simulink model "SPMe_ESC_validation_simulink"  (R2024a)
settings: Solver=FixedStepAuto  StartTime=0.0  StopTime=t_end  FixedStep=param.dt  MaxStep=1  RelTol=1e-6
values from neighbouring files (symbols this model uses):
  R_esc = R_escs(param.soc_name)    [SPMe_EqCM_ESC_validation.m]    (also in run_SPMe_ESC_validation.m = 0.0067; run_parallel_SPMe_ESC.m = 0.0134)
  R_tab = R_tabs(param.soc_name)    [SPMe_EqCM_ESC_validation.m]    (also in run_SPMe_ESC_validation.m = 0.0086; run_parallel_SPMe_ESC.m = 0.0172)
  V_min = 0    [SPMe_EqCM_ESC_validation.m]    (also in run_SPMe_ESC_validation.m; run_parallel_SPMe_ESC.m)
libraries: eeGeneralControl x1, simulink x1
settings Model: Creator=tom  LastModifiedBy=Vivian
settings SolverCC: AlgebraicLoopSolver=TrustRegion
settings DebuggingCC: UnconnectedInputMsg=warning  UnconnectedOutputMsg=warning  UnconnectedLineMsg=warning
settings ModelReferenceCC: EnableRefExpFcnMdlSchedulingChecks=on
settings RTWCC: GPUComputeCapability=3.5  DLArmComputeVersion=19.05

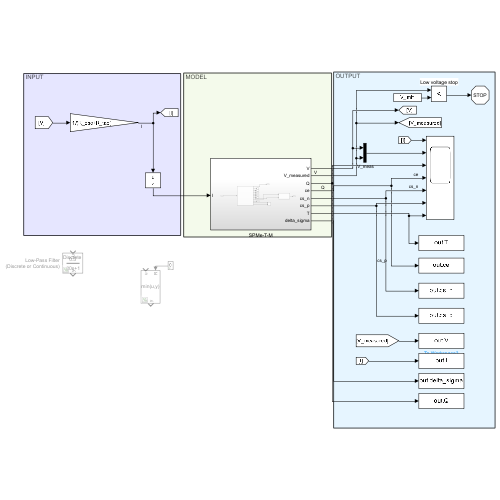
[thumbnail: Simulink's stored preview of the top-level diagram]
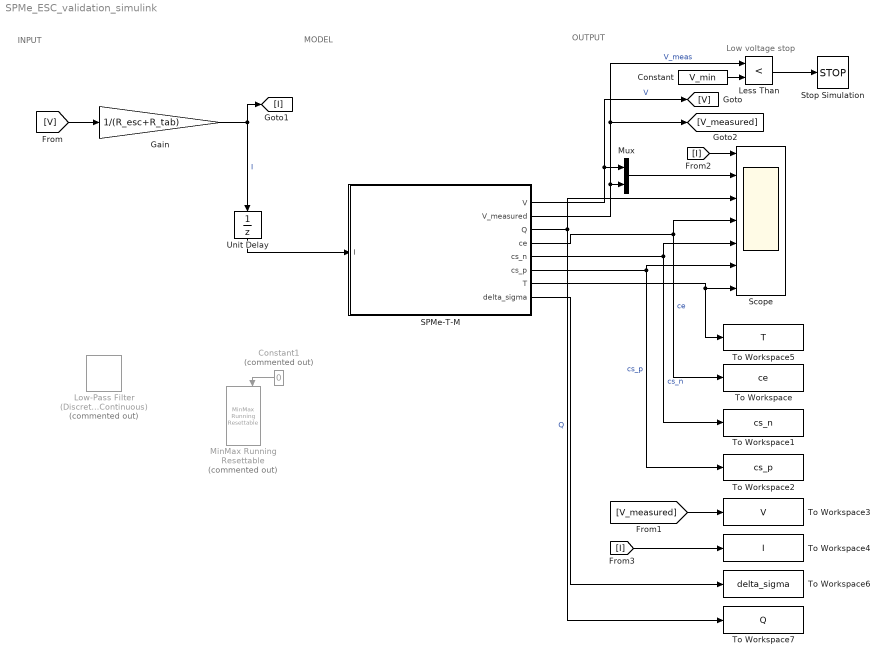
== system SPMe_ESC_validation_simulink ==
  note: OUTPUT
  note: MODEL
  note: INPUT
  note: Low voltage stop
  Constant : Constant  Value=V_min
  Constant1 : Constant  Commented=on  Value=0
  Gain : Gain  Gain=1/(R_esc+R_tab)
  Less Than : RelationalOperator  Operator=<  OutDataTypeStr=boolean  RndMeth=Simplest  InputSameDT=off
  Low-Pass Filter (Discrete or Continuous) : eeGeneralControl/Low-Pass Filter (Discrete or Continuous)  Commented=on  K=0.5  T=20  B=inf  A=-inf  init_option=Inherited from block input  x0=0  Ts=-1
  MinMax Running Resettable : simulink/Math Operations/MinMax Running Resettable  Commented=on  Function=min  vinit=1000
  Mux : Mux  Inputs=2
  SPMe-T-M : Subsystem
  Scope : Scope  NumInputPorts=7
  Stop Simulation : Stop
  To Workspace : ToWorkspace  VariableName=ce  SaveFormat=Timeseries  SampleTime=-1
  To Workspace1 : ToWorkspace  VariableName=cs_n  SaveFormat=Timeseries  SampleTime=-1
  To Workspace2 : ToWorkspace  VariableName=cs_p  SaveFormat=Timeseries  SampleTime=-1
  To Workspace3 : ToWorkspace  VariableName=V  SaveFormat=Timeseries  SampleTime=-1
  To Workspace4 : ToWorkspace  VariableName=I  SaveFormat=Timeseries  SampleTime=-1
  To Workspace5 : ToWorkspace  VariableName=T  SaveFormat=Timeseries  SampleTime=-1
  To Workspace6 : ToWorkspace  VariableName=delta_sigma  SaveFormat=Timeseries  SampleTime=-1
  To Workspace7 : ToWorkspace  VariableName=Q  SaveFormat=Timeseries  SampleTime=-1
  Unit Delay : UnitDelay  SampleTime=-1  HasFrameUpgradeWarning=on
  wires:
  SPMe-T-M/3(Q) -> To Workspace7/1, Scope/3  "Q"
  SPMe-T-M/5(cs_n) -> Scope/5, To Workspace1/1  "cs_n"
  SPMe-T-M/6(cs_p) -> Scope/6, To Workspace2/1  "cs_p"
  Less Than/1 -> Stop Simulation/1
  Constant/1 -> Less Than/2
  SPMe-T-M/4(ce) -> To Workspace/1, Scope/4  "ce"
  SPMe-T-M/1(V) -> [V], Mux/1  "V"
  SPMe-T-M/2(V_measured) -> Less Than/1, [V_measured], Mux/2  "V_meas"
  Gain/1 -> Unit Delay/1, [I]  "I"
  Mux/1 -> Scope/2
  [V_measured] -> To Workspace3/1
  [I] -> Scope/1
  [I] -> To Workspace4/1
  SPMe-T-M/7(T) -> To Workspace5/1, Scope/7
  [V] -> Gain/1
  SPMe-T-M/8(delta_sigma) -> To Workspace6/1
  Unit Delay/1 -> SPMe-T-M/1(I)
  Constant1/1 -> MinMax Running Resettable/2

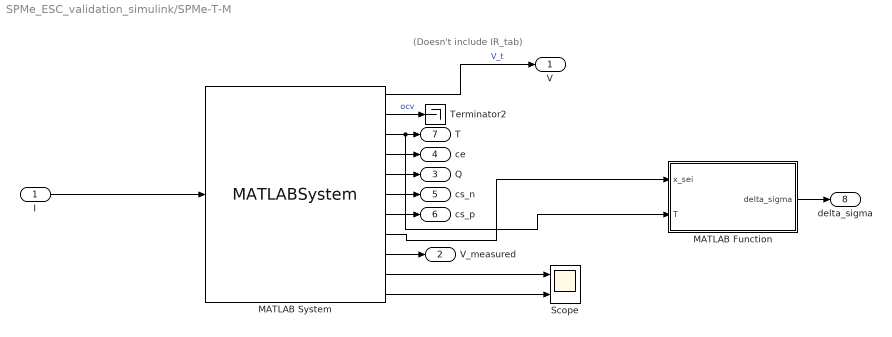
== system SPMe_ESC_validation_simulink/SPMe-T-M ==
  note: (Doesn't include IR_tab)
  I : Inport
  MATLAB Function : MATLAB Function  TreatAsAtomicUnit=on
  MATLAB System : MATLABSystem  System=pybamm_bat  SimulateUsing=Interpreted execution
      mask Type: pybamm_bat
      mask Display:
      | disp('pybamm_bat');
      | port_label('input',1,'current');
      | port_label('output',1,'V_t');
      | port_label('output',2,'ocv');
      | port_label('output',3,'T');
      | port_label('output',4,'ce');
      | port_label('output',5,'heating');
      | port_label('output',6,'neg_conc');
      | port_label('output',7,'pos_conc');
      | port_label('output',8,'x_sei');
      | port_label('output',9,'V_meas');
      | port_label('output',10,'ocp_n');
      | port_label('output',11,'ocp_p');
  Scope : Scope  NumInputPorts=2
  Terminator2 : Terminator
  V : Outport
  V_measured : Outport  Port=2
  Q : Outport  Port=3  VectorParamsAs1DForOutWhenUnconnected=off
  ce : Outport  Port=4
  cs_n : Outport  Port=5  VectorParamsAs1DForOutWhenUnconnected=off
  cs_p : Outport  Port=6  VectorParamsAs1DForOutWhenUnconnected=off
  T : Outport  Port=7
  delta_sigma : Outport  Port=8
  wires:
  MATLAB System/4 -> ce/1
  MATLAB System/5 -> Q/1
  MATLAB System/6 -> cs_n/1
  MATLAB System/7 -> cs_p/1
  MATLAB System/1 -> V/1  "V_t"
  MATLAB System/8 -> MATLAB Function/1(x_sei)
  MATLAB System/9 -> V_measured/1
  MATLAB System/3 -> MATLAB Function/2(T), T/1
  MATLAB System/2 -> Terminator2/1  "ocv"
  MATLAB Function/1(delta_sigma) -> delta_sigma/1
  I/1 -> MATLAB System/1
  MATLAB System/10 -> Scope/1
  MATLAB System/11 -> Scope/2

== matlab function SPMe_ESC_validation_simulink/SPMe-T-M/MATLAB Function ==
  data: x_sei input; delta_sigma output; T input
function delta_sigma  = expansion(x_sei, T)
%XSEI2PTOTAL 
% Mechanical params
M_C6 = 72/1000; %kg/mol
% V_head_0 = 6.65e-6; %m3 (0.121*0.074*0.0055)*0.135
% L = 2.4/1000; %m
% E = 0.19e6; %Pa
% alpha_cell = 1.1e-6; %m/K
% P_atm = 101; %kPa
% P_crit = 158.7731; %kPa
R = 8.3145; %J.mol-1.K-1
A = 0.009; %m2 (0.121*0.074)
DMC = [6.4338; 1413; -44.25]; %Antoine coeffs [A B C] 
EC = [6.4897; 1836.57; -102.23];
y_dmc = 0.7;
y_ec = 1-y_dmc;         
m_an = 0.0191; 
x_sei_0 = 0.15;
% T_amb = 273.15+25; % K
% sigma_0 = 1.5120e+04;

% Internal cell pressure
V_head_0 = 6.65e-06; %m-3
L_p0 = 2.4e-3; %m for 2 poron
E_p = 0.19e6; %Pa Young's modulus for poron
% E_c = 1e12; %assume large by default
alpha = 1.1e-6; %m/K
P_atm = 101e3; %Pa
% P_crit = 158e3; %Pa
% P0 = 14e3; %Pa
R = 8.3145; %J.mol-1.K-1
% k_b = 1.380649e-23; %m2.kg.s-2.K-1;
T_amb = 273.15+25; % K
sigma_0 = 1.5120e+04;
% L_cs0 = 5.5e-3; %m initial cell solid thickness
% V_cell = 0.130*0.089*0.055; % [130mm×89mm×5.5mm] active material

% P_elyte
Psat_EC = 10.^(EC(1)-EC(2)./(EC(3)+T));
Psat_DMC = 10.^(DMC(1)-DMC(2)./(DMC(3)+T)); 
P_elyte = (y_dmc*Psat_DMC + y_ec*Psat_EC)*1e3; 

% P_CO2
n_CO2 = 0.5*m_an/M_C6*(x_sei_0-x_sei);

% Solve for gas volume and pressure
delta_sigma_calc = P_elyte - sigma_0 - P_atm;
a = 1;
b = -(V_head_0 + A.*(L_p0/E_p*(delta_sigma_calc) - alpha.*(T-T_amb)));
c = -A*L_p0/E_p.*n_CO2.*R.*(T);
V_g0 = (-b+sqrt(max(b.^2-4.*a.*c,0)))/(2*a);
V_g = max(V_g0, V_head_0); % min V_g = V_head_0

P_CO2 = n_CO2.*R.*T./V_g;
P_gas = P_elyte + P_CO2;

delta_sigma = max(P_gas-P_atm-sigma_0, E_p./L_p0.*alpha.*(T-T_amb));
end
